simulink model "sampleModel1779"  (R2023a)
settings: Solver=VariableStepAuto  StartTime=0.0  StopTime=10.0  RelTol=1e-3
libraries: hdlsllib x5
settings Model: Creator=user1  LastModifiedBy=user1

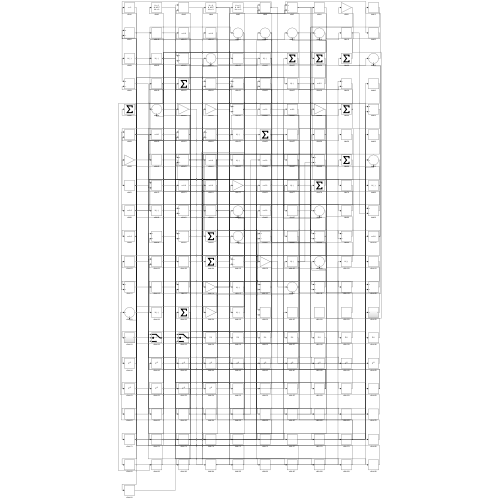
[thumbnail: Simulink's stored preview of the top-level diagram]
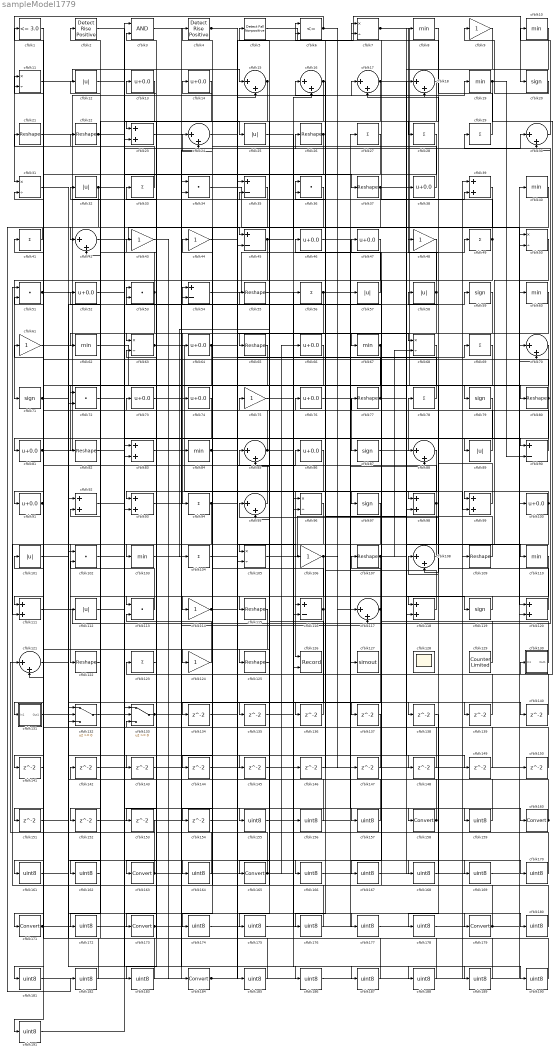
== system sampleModel1779 ==
  cfblk1 : hdlsllib/Logic and Bit Operations/Compare To Constant  relop=<=  const=3.0  OutDataTypeStr=boolean
  cfblk{8,10,19,40,60,62,67,84,103,110} (10 alike) : MinMax
  cfblk{13..14,38,46..47,52,64,66,73..74,76,81,86,91,100} (15 alike) : Bias  Bias=0.0  SaturateOnIntegerOverflow=off
  cfblk{12,25,32,57..58,89,101,112} (8 alike) : Abs  SaturateOnIntegerOverflow=off
  cfblk{34,36,51,53,72,102,113} (7 alike) : DotProduct  OutDataTypeStr=Inherit: Inherit via internal rule
  cfblk{27..29,33,41,49,56,69,78,94,104,123} (12 alike) : Sum  Inputs=+
  cfblk{7,11,31,50,63,68,96,105} (8 alike) : Product  Inputs=*/  RndMeth=Zero  SaturateOnIntegerOverflow=on
  cfblk{9,43..44,48,61,75,106,114,124} (9 alike) : Gain
  cfblk{21..22,26,37,55,65,77,80,82,107,109,115,122,125} (14 alike) : Reshape
  cfblk{15..18,24,30,42,70,85,88,95,108,117,121} (14 alike) : Sum  Inputs=|++
  cfblk{23,39,83,92..93,98..99,111,118,120} (10 alike) : Sum
  cfblk{35,45,54,90,116} (5 alike) : Sum  Inputs=+-
  cfblk{20,59,71,79,87,97,119} (7 alike) : Signum
  cfblk126 : Record  FileSettingsInternal="{\"entries\":[{\"content\":{\"excelSettings\":{\"content\":{},\"type\":\"Streamout.ExcelSettings\"}},\"type\":\"Streamout.FileSettingStorage\",\"uuid\":\"\"}],\"packageUris\":[\"http:\\/\\/schema.mathworks.com\\/mf0\\/streamout_blocks\\/R2020a\"],\"version\":\"1.0\"}"  Layout=[1 1]  SignalsInternal="{\"entries\":[{\"content\":{\"signals\":[{\"content\":{\"blockPath\":[],\"dimensions\":[1],\"domain\":\"\",\"lineColor\":\"#a2142f\",\"plots\":[1],\"port\":1,\"signalID\":3981,\"signalName\":\"XY Graph:1\"},\"type\":\"RecordBlkView.Signal\",\"uuid\":\"\"},{\"content\":{\"blockPath\":[],\"dimensions\":[1],\"domain\":\"\",\"lineColor\":\"#139fff\",\"plots\":[1],\"port\":2,\"signalID\":3984,\"signalName\":\"XY Graph:2\"},\"type\":\"RecordBlkView.Signal\",\"uuid\":\"\"}]},\"type\":\"RecordBlkView.InputSignals\",\"uuid\":\"\"}],\"packageUris\":[\"http:\\/\\/schema.mathworks.com\\/mf0\\/streamout_blocks\\/R2020a\"],\"version\":\"1.0\"}"  VisualizationBindings="{\"xyplotplugin\":{\"info\":[{\"series\":[{\"bindingParametersList\":[{\"parameter\":\"X-Axis\",\"signalID\":3981,\"signalName\":\"XY Graph:1\"},{\"parameter\":\"Y-Axis\",\"signalID\":3984,\"signalName\":\"XY Graph:2\"}],\"seriesID\":50670}],\"subplotID\":1}]}}"  CompatibilityTag=XY  st=-1
  cfblk127 : ToWorkspace  VariableName=simout  SaveFormat=Timeseries  SampleTime=-1
  cfblk128 : Scope
      settings: Floating=on
  cfblk129 : hdlsllib/Sources/Counter Limited  uplimit=7  tsamp=-1
  cfblk130 : Subsystem
      settings: LibrarySourceBlock=|
      | hdlsllib/Ports &
      | Subsystems/Subsystem
  cfblk131 : Subsystem
      settings: LibrarySourceBlock=|
      | hdlsllib/Ports &
      | Subsystems/Subsystem
  cfblk132 : Switch  SaturateOnIntegerOverflow=off  InputSameDT=off
  cfblk133 : Switch  SaturateOnIntegerOverflow=off  InputSameDT=off
  cfblk{134..154} (21 alike) : Delay  SampleTime=1
  cfblk{155..157,159,161..162,164,166..170,172,174..178,180..183,185..191} (29 alike) : DataTypeConversion  OutDataTypeStr=uint8  SaturateOnIntegerOverflow=off  RndMeth=Floor
  cfblk{158,160,163,165,171,173,179,184} (8 alike) : DataTypeConversion  SaturateOnIntegerOverflow=off  RndMeth=Floor
  cfblk2 : hdlsllib/Logic and Bit Operations/Detect Rise Positive  vinit=0  OutDataTypeStr=boolean
  cfblk3 : Logic  AllPortsSameDT=off  OutDataTypeStr=boolean
  cfblk4 : hdlsllib/Logic and Bit Operations/Detect Rise Positive  vinit=0  OutDataTypeStr=boolean
  cfblk5 : hdlsllib/Logic and Bit Operations/Detect Fall Nonpositive  vinit=0  OutDataTypeStr=boolean
  cfblk6 : RelationalOperator  Operator=<=  OutDataTypeStr=boolean  InputSameDT=off
  wires:
  cfblk59/1 -> cfblk94/1
  cfblk11/1 -> cfblk15/1
  cfblk61/1 -> cfblk54/1
  cfblk42/1 -> cfblk45/1
  cfblk106/1 -> cfblk117/1, cfblk162/1
  cfblk26/1 -> cfblk104/1, cfblk131/1(In1)
  cfblk50/1 -> cfblk113/1
  cfblk81/1 -> cfblk17/1, cfblk55/1
  cfblk119/1 -> cfblk118/1
  cfblk53/1 -> cfblk32/1, cfblk62/1
  cfblk24/1 -> cfblk179/1
  cfblk6/1 -> cfblk31/1, cfblk147/1
  cfblk21/1 -> cfblk19/1
  cfblk56/1 -> cfblk98/1, cfblk112/1, cfblk88/2
  cfblk111/1 -> cfblk29/1
  cfblk117/1 -> cfblk115/1, cfblk132/3
  cfblk47/1 -> cfblk71/1
  cfblk63/1 -> cfblk126/1, cfblk35/2
  cfblk129/1 -> cfblk53/1
  cfblk38/1 -> cfblk14/1
  cfblk93/1 -> cfblk117/2
  cfblk107/1 -> cfblk119/1, cfblk68/2, cfblk144/1
  cfblk7/1 -> cfblk80/1, cfblk110/1
  cfblk57/1 -> cfblk46/1
  cfblk78/1 -> cfblk4/1
  cfblk123/1 -> cfblk163/1
  cfblk5/1 -> cfblk20/1
  cfblk16/1 -> cfblk103/1, cfblk136/1
  cfblk124/1 -> cfblk73/1
  cfblk130/1(Out1) -> cfblk58/1
  cfblk20/1 -> cfblk9/1
  cfblk32/1 -> cfblk81/1, cfblk39/2
  cfblk17/1 -> cfblk23/1, cfblk140/1
  cfblk28/1 -> cfblk105/1
  cfblk40/1 -> cfblk65/1
  cfblk2/1 -> cfblk158/1
  cfblk89/1 -> cfblk61/1
  cfblk37/1 -> cfblk124/1, cfblk99/2
  cfblk49/1 -> cfblk67/1, cfblk7/1
  cfblk31/1 -> cfblk79/1
  cfblk100/1 -> cfblk99/1, cfblk30/2, cfblk111/2
  cfblk90/1 -> cfblk22/1
  cfblk27/1 -> cfblk171/1
  cfblk58/1 -> cfblk8/1, cfblk63/1
  cfblk104/1 -> cfblk69/1
  cfblk66/1 -> cfblk91/1
  cfblk95/1 -> cfblk33/1
  cfblk94/1 -> cfblk122/1, cfblk7/2, cfblk154/1
  cfblk54/1 -> cfblk49/1
  cfblk120/1 -> cfblk95/1
  cfblk77/1 -> cfblk6/1, cfblk149/1
  cfblk10/1 -> cfblk118/2
  cfblk114/1 -> cfblk59/1, cfblk86/1
  cfblk33/1 -> cfblk21/1
  cfblk118/1 -> cfblk16/1
  cfblk9/1 -> cfblk98/2
  cfblk112/1 -> cfblk26/1
  cfblk116/1 -> cfblk44/1, cfblk183/1
  cfblk67/1 -> cfblk82/1, cfblk116/2
  cfblk108/1 -> cfblk76/1
  cfblk87/1 -> cfblk78/1
  cfblk97/1 -> cfblk116/1
  cfblk85/1 -> cfblk13/1, cfblk170/1
  cfblk62/1 -> cfblk126/2
  cfblk102/1 -> cfblk160/1
  cfblk71/1 -> cfblk143/1, cfblk161/1
  cfblk12/1 -> cfblk89/1
  cfblk80/1 -> cfblk31/2, cfblk132/2
  cfblk69/1 -> cfblk108/2
  cfblk76/1 -> cfblk87/1
  cfblk96/1 -> cfblk173/1
  cfblk36/1 -> cfblk64/1
  cfblk19/1 -> cfblk130/1(In1), cfblk90/2
  cfblk51/1 -> cfblk18/1, cfblk168/1
  cfblk132/1 -> cfblk23/2
  cfblk29/1 -> cfblk6/2
  cfblk101/1 -> cfblk53/2
  cfblk113/1 -> cfblk52/1
  cfblk84/1 -> cfblk106/1, cfblk166/1
  cfblk99/1 -> cfblk17/2
  cfblk15/1 -> cfblk45/2, cfblk42/2
  cfblk43/1 -> cfblk184/1
  cfblk18/1 -> cfblk125/1
  cfblk105/1 -> cfblk88/1
  cfblk30/1 -> cfblk10/1
  cfblk8/1 -> cfblk28/1
  cfblk4/1 -> cfblk90/1, cfblk68/1
  cfblk91/1 -> cfblk181/1, cfblk191/1
  cfblk64/1 -> cfblk84/1, cfblk133/2, cfblk97/1, cfblk152/1
  cfblk133/1 -> cfblk74/1, cfblk148/1
  cfblk72/1 -> cfblk30/1
  cfblk74/1 -> cfblk111/1
  cfblk45/1 -> cfblk16/2, cfblk72/2
  cfblk122/1 -> cfblk12/1
  cfblk86/1 -> cfblk93/1
  cfblk14/1 -> cfblk42/1
  cfblk65/1 -> cfblk93/2
  cfblk22/1 -> cfblk37/1, cfblk25/1
  cfblk34/1 -> cfblk120/1
  cfblk35/1 -> cfblk114/1
  cfblk98/1 -> cfblk11/1, cfblk137/1
  cfblk109/1 -> cfblk36/1
  cfblk125/1 -> cfblk85/1
  cfblk1/1 -> cfblk121/2
  cfblk68/1 -> cfblk72/1
  cfblk60/1 -> cfblk165/1
  cfblk88/1 -> cfblk134/1
  cfblk134/1 -> cfblk105/2
  cfblk103/1 -> cfblk135/1
  cfblk136/1 -> cfblk95/2
  cfblk137/1 -> cfblk133/3
  cfblk73/1 -> cfblk138/1
  cfblk23/1 -> cfblk139/1
  cfblk139/1 -> cfblk108/1
  cfblk140/1 -> cfblk63/2
  cfblk39/1 -> cfblk141/1
  cfblk141/1 -> cfblk1/1
  cfblk142/1 -> cfblk120/2
  cfblk144/1 -> cfblk50/1
  cfblk131/1(Out1) -> cfblk145/1
  cfblk146/1 -> cfblk36/2
  cfblk147/1 -> cfblk54/2
  cfblk148/1 -> cfblk85/2
  cfblk149/1 -> cfblk18/2
  cfblk150/1 -> cfblk51/2
  cfblk115/1 -> cfblk151/1
  cfblk152/1 -> cfblk34/2
  cfblk110/1 -> cfblk153/1
  cfblk153/1 -> cfblk121/1
  cfblk154/1 -> cfblk35/1
  cfblk3/1 -> cfblk155/1
  cfblk155/1 -> cfblk57/1
  cfblk25/1 -> cfblk156/1
  cfblk156/1 -> cfblk3/1
  cfblk143/1 -> cfblk157/1
  cfblk157/1 -> cfblk3/2
  cfblk158/1 -> cfblk107/1, cfblk132/1, cfblk47/1
  cfblk46/1 -> cfblk159/1
  cfblk159/1 -> cfblk2/1
  cfblk160/1 -> cfblk142/1, cfblk39/1
  cfblk161/1 -> cfblk102/1
  cfblk162/1 -> cfblk102/2
  cfblk163/1 -> cfblk11/2, cfblk56/1
  cfblk52/1 -> cfblk164/1
  cfblk164/1 -> cfblk123/1
  cfblk165/1 -> cfblk113/2, cfblk66/1
  cfblk166/1 -> cfblk60/1
  cfblk48/1 -> cfblk167/1
  cfblk167/1 -> cfblk38/1
  cfblk168/1 -> cfblk48/1
  cfblk75/1 -> cfblk169/1
  cfblk169/1 -> cfblk100/1
  cfblk170/1 -> cfblk75/1
  cfblk171/1 -> cfblk34/1, cfblk127/1
  cfblk13/1 -> cfblk172/1
  cfblk172/1 -> cfblk27/1
  cfblk173/1 -> cfblk146/1, cfblk50/2
  cfblk79/1 -> cfblk174/1
  cfblk174/1 -> cfblk96/1
  cfblk145/1 -> cfblk175/1
  cfblk175/1 -> cfblk96/2
  cfblk70/1 -> cfblk176/1
  cfblk176/1 -> cfblk51/1
  cfblk121/1 -> cfblk177/1
  cfblk177/1 -> cfblk70/1
  cfblk138/1 -> cfblk178/1
  cfblk178/1 -> cfblk70/2
  cfblk179/1 -> cfblk150/1, cfblk77/1, cfblk5/1
  cfblk55/1 -> cfblk180/1
  cfblk180/1 -> cfblk24/1
  cfblk181/1 -> cfblk24/2
  cfblk41/1 -> cfblk182/1
  cfblk182/1 -> cfblk101/1
  cfblk183/1 -> cfblk41/1
  cfblk184/1 -> cfblk15/2, cfblk40/1
  cfblk44/1 -> cfblk185/1
  cfblk185/1 -> cfblk43/1
  cfblk92/1 -> cfblk186/1
  cfblk186/1 -> cfblk109/1
  cfblk82/1 -> cfblk187/1
  cfblk187/1 -> cfblk92/1
  cfblk151/1 -> cfblk188/1
  cfblk188/1 -> cfblk92/2
  cfblk83/1 -> cfblk189/1
  cfblk189/1 -> cfblk133/1
  cfblk135/1 -> cfblk190/1
  cfblk190/1 -> cfblk83/1
  cfblk191/1 -> cfblk83/2

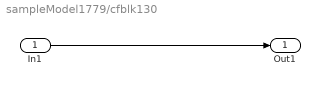
== system sampleModel1779/cfblk130 ==
  In1 : Inport
  Out1 : Outport
  wires:
  In1/1 -> Out1/1

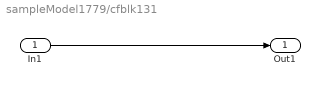
== system sampleModel1779/cfblk131 ==
  In1 : Inport
  Out1 : Outport
  wires:
  In1/1 -> Out1/1
